simulink model "QuedaLivre"  (R2020a)
settings: Solver=VariableStepAuto  StartTime=0.0  StopTime=10.0  RelTol=1e-3
values from neighbouring files (symbols this model uses):
  b = 0.3    [Queda_livre.m]
  m = 5    [Queda_livre.m]
settings Model: Creator=gabri  LastModifiedBy=gabri

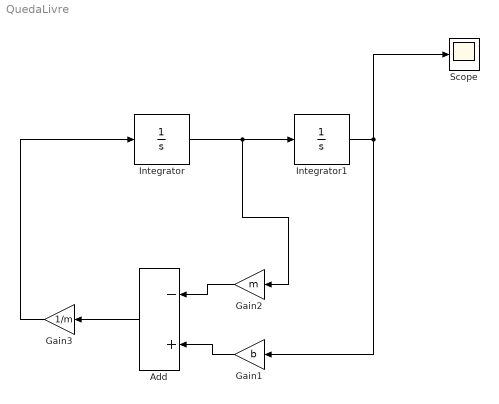
== system QuedaLivre ==
  Add : Sum  Inputs=-+
  Gain1 : Gain  Gain=b
  Gain2 : Gain  Gain=m
  Gain3 : Gain  Gain=1/m
  Integrator : Integrator
  Integrator1 : Integrator  InitialCondition=1
  Scope : Scope
  wires:
  Integrator/1 -> Gain2/1, Integrator1/1
  Integrator1/1 -> Gain1/1, Scope/1
  Gain2/1 -> Add/1
  Gain1/1 -> Add/2
  Add/1 -> Gain3/1
  Gain3/1 -> Integrator/1
